simulink model "high_gain"  (R2023a)
settings: Solver=VariableStepAuto  StartTime=0.0  StopTime=10.0  RelTol=1e-3
settings Model: Creator=belov  LastModifiedBy=belov

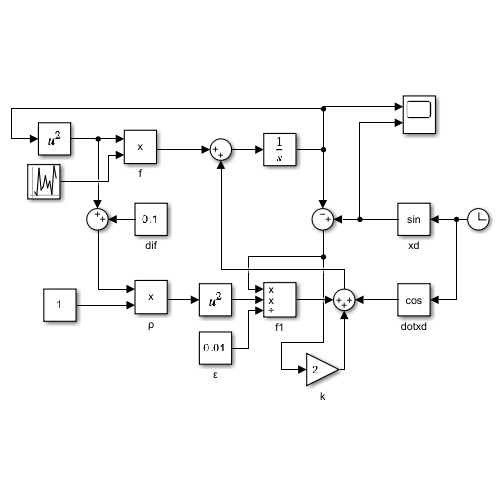
[thumbnail: Simulink's stored preview of the top-level diagram]
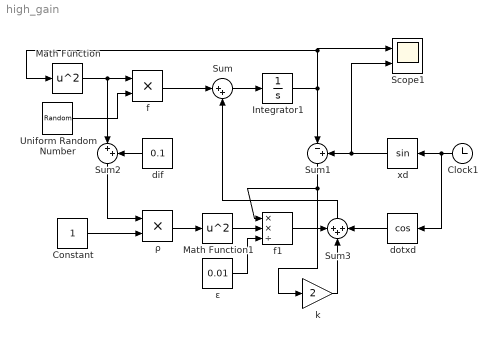
== system high_gain ==
  Clock1 : Clock
  Constant : Constant
  Integrator1 : Integrator  InitialCondition=1
  Math Function : Math  Operator=square
  Math Function1 : Math  Operator=square
  Scope1 : Scope  NumInputPorts=2
  Sum : Sum  Inputs=|++
  Sum1 : Sum  Inputs=|-+
  Sum2 : Sum  Inputs=|++
  Sum3 : Sum  Inputs=+++
  Uniform Random Number : UniformRandomNumber  SampleTime=0.1
  dif : Constant  Value=0.1
  dotxd : Trigonometry  Operator=cos
  f : Product  Inputs=**
  f1 : Product  Inputs=**/
  k : Gain  Gain=2
  xd : Trigonometry
  ε : Constant  Value=0.01
  ρ : Product  Inputs=**
  wires:
  Sum/1 -> Integrator1/1
  Integrator1/1 -> Sum1/1, Math Function/1, Scope1/1
  Clock1/1 -> dotxd/1, xd/1
  Math Function/1 -> f/1, Sum2/1
  f/1 -> Sum/1
  xd/1 -> Scope1/2, Sum1/2
  Uniform Random Number/1 -> f/2
  Constant/1 -> ρ/2
  Sum2/1 -> ρ/1
  dif/1 -> Sum2/2
  ρ/1 -> Math Function1/1
  Math Function1/1 -> f1/2
  ε/1 -> f1/3
  Sum1/1 -> k/1, f1/1
  f1/1 -> Sum3/1
  dotxd/1 -> Sum3/3
  k/1 -> Sum3/2
  Sum3/1 -> Sum/2
